simulink model "untitled"  (R2023b)
settings: Solver=FixedStepAuto  StartTime=0.0  StopTime=20  FixedStep=1e-5  MinStep=1e-6  RelTol=1e-3  AbsTol=1e-3
libraries: C_uF_lib x4, nesl_utility x2, SignalEditorBlockLib x1
settings Model: Creator=malli  LastModifiedBy=mavap
settings SolverCC: AutoScaleAbsTol=off  InitialStep=1e-6  MaxConsecutiveMinStep=1000000  AlgebraicLoopSolver=TrustRegion  SolverResetMethod=Robust  EnableFixedStepZeroCrossing=on  MaxZcPerStep=1
settings DataIOCC: MaxDataPoints=1000000  InspectSignalLogs=on
settings DebuggingCC: UnconnectedInputMsg=warning  UnconnectedOutputMsg=warning  UnconnectedLineMsg=warning  SymbolicDimsDataTypeCodeGenerationDiagnostic=none
settings HardwareCC: ProdBitPerLong=64  ProdHWDeviceType=Intel->x86-64 (Linux 64)
settings ModelReferenceCC: EnableRefExpFcnMdlSchedulingChecks=on
settings SFSimCC: CustomCodeUndefinedFunction=UseInterfaceOnly
settings RTWCC: DLArmComputeVersion=19.05
settings SimscapeCC: SimscapeNormalizeSystem=off  SimscapeLogType=all  SimscapeLogSimulationStatistics=on  SimscapeLogToSDI=on  SimscapeLogLimitData=off  SimscapeLogDataHistory=10000000

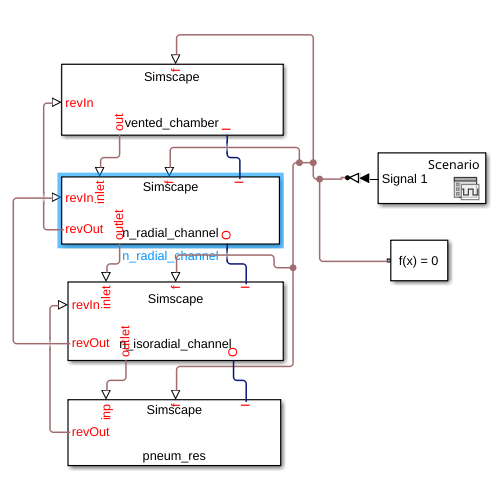
[thumbnail: Simulink's stored preview of the top-level diagram]
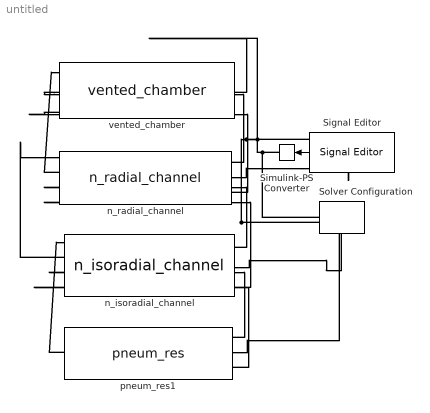
== system untitled ==
  Signal Editor : SignalEditorBlockLib/Signal Editor  FileName=/home/mavap/Documents/MATLAB/C_uF_lumped/Velocity profiles/up10down10.mat  ActiveScenario=Scenario  ActiveSignal=Signal 1  IsBus=off  OutputBusObjectStr=Bus: BusObject  SampleTime=0.00001  ZeroCross=off  OutputAfterFinalValue=Extrapolation  Unit=Hz  PreserveSignalName=on  ApplySigPropsToAllScenarios=on  ApplySigPropsToAllSignals=off
  Simulink-PS Converter : nesl_utility/Simulink-PS Converter  PhysicalDomain=network_engine_domain  SubClassName=ps_input  LeftPortType=input  RightPortType=output  PseudoPeriodic=off  Frequencies=[]  NoiseDistribution=none  NoiseParameters=[]  Unit=Hz  AffineConversion=on  FilteringAndDerivatives=filter  SimscapeFilterOrder=1  InputFilterTimeConstant=0.00001  UdotUserProvided=0
  Solver Configuration : nesl_utility/Solver Configuration  PhysicalDomain=network_engine_domain  SubClassName=solver  LeftPortType=input  RightPortType=generic  Tones=[]  Harmonics=[]  SimulateNoise=off  Profile=off  UseLocalSampling=off  EnableSwitchedLinearOptims=on  FrequencyDomain=off  UseCCode=off  RelTol=0.001  AbsTol=0.001  MinStep=1e-09  ToWorkspace=off  RevertToSquareIcSolve=off  NumHomotopyIterations=100  PhasorMode=off  PhasorModeNumHarmonics=1  ConsistencySolver=NEWTON_XTOL_AFTER_FTOL  IndexReductionMethod=DerivativeReplacement  DoDC=on  ResidualTolerance=1e-09  ConsistencyTolSource=GLOBAL  ConsistencyAbsTol=0.001  ConsistencyRelTol=0.001  ConsistencyTolFactor=0.000001  UseLocalSolver=off  LocalSolverChoice=NE_BACKWARD_EULER_ADVANCER  ResolveIndetEquations=on  FunctionEvalNumThread=1  LocalSolverSampleTime=0.001  DoFixedCost=off  MaxNonlinIter=3  MaxModeIter=2  ComputeImpulses=off  ImpulseIterations=2  LinearAlgebra=auto  LinearAlgebraNumThread=0  EquationFormulation=NE_TIME_EF  DelaysMemoryBudget=1024  AutomaticFiltering=on  FilteringTimeConstant=0.00001  PartitionStorageMethod=AS_NEEDED  PartitionMemoryBudget=1024  PartitionMethod=ROBUST  MultibodyUseLocalSolver=off  MultibodyLocalSolverChoice=ODE1  MultibodyLocalSolverSampleTime=0.001
  n_isoradial_channel : C_uF_lib/n_isoradial_channel  w=2 mm  d=40 um  l=20 mm  r=70 mm  init_fill=0  theta=pi/2  dir=-1  q_specify=off  q_priority=None  q=0 mm^3/s  q_nominal_specify=off  q_nominal_unit=mm^3/s  q_nominal_value=1  q_dot_specify=off  q_dot_priority=None  q_dot=0 mm^3/s^2  q_dot_nominal_specify=off  q_dot_nominal_unit=mm^3/s^2  q_dot_nominal_value=1  f_dot_specify=off  f_dot_priority=None  f_dot=0 Hz/s  f_dot_nominal_specify=off  f_dot_nominal_unit=Hz/s  f_dot_nominal_value=1  p_specify=off  p_priority=None  p=0 Pa  p_nominal_specify=off  p_nominal_unit=Pa  p_nominal_value=1  fill_specify=off  fill_priority=None  fill=0  fill_nominal_specify=off  fill_nominal_unit=1  fill_nominal_value=1  V_liquid_specify=off  V_liquid_priority=None  V_liquid=0 mm^3  V_liquid_nominal_specify=off  V_liquid_nominal_unit=mm^3  V_liquid_nominal_value=1  InO_specify=off  InO_priority=None  InO=0  InO_nominal_specify=off  InO_nominal_unit=1  InO_nominal_value=1  p_IRRF_specify=off  p_IRRF_priority=None  p_IRRF=0 Pa  p_IRRF_nominal_specify=off  p_IRRF_nominal_unit=Pa  p_IRRF_nominal_value=1  p_Euler_specify=off  p_Euler_priority=None  p_Euler=0 Pa  p_Euler_nominal_specify=off  p_Euler_nominal_unit=Pa  p_Euler_nominal_value=1  p_visc_specify=off  p_visc_priority=None  p_visc=0 Pa  p_visc_nominal_specify=off  p_visc_nominal_unit=Pa  p_visc_nominal_value=1  p_cap_specify=off  p_cap_priority=None  p_cap=0 Pa  p_cap_nominal_specify=off  p_cap_nominal_unit=Pa  p_cap_nominal_value=1  wet_specify=off  wet_priority=None  wet=0  wet_nominal_specify=off  wet_nominal_unit=1  wet_nominal_value=1
      settings: InternalSimscapePortConfiguration="{\"Bottom\":[{\"id\":\"O\",\"label\":\"O\",\"type\":\"C_uF.C_uF\"},{\"id\":\"outlet\",\"label\":\"outlet\",\"type\":\"output\"}],\"Left\":[],\"Right\":[{\"id\":\"revIn\",\"label\":\"revIn\",\"type\":\"input\"},{\"id\":\"revOut\",\"label\":\"revOut\",\"type\":\"output\"}],\"Top\":[{\"id\":\"I\",\"label\":\"I\",\"type\":\"C_uF.C_uF\"},{\"id\":\"f\",\"label\":\"f\",\"type\":\"input\"},{\"id\":\"inlet\",\"label\":\"inlet\",\"type\":\"input\"}]}"
  n_radial_channel : C_uF_lib/n_radial_channel  w=2 mm  d=40 um  r_in=20 mm  r_out=70 mm  init_fill=0  theta=pi/2  q_specify=off  q_priority=None  q=0 mm^3/s  q_nominal_specify=off  q_nominal_unit=mm^3/s  q_nominal_value=1  q_dot_specify=off  q_dot_priority=None  q_dot=0 mm^3/s^2  q_dot_nominal_specify=off  q_dot_nominal_unit=mm^3/s^2  q_dot_nominal_value=1  p_specify=off  p_priority=None  p=0 Pa  p_nominal_specify=off  p_nominal_unit=Pa  p_nominal_value=1  fill_specify=off  fill_priority=None  fill=0  fill_nominal_specify=off  fill_nominal_unit=1  fill_nominal_value=1  V_liquid_specify=off  V_liquid_priority=None  V_liquid=0 mm^3  V_liquid_nominal_specify=off  V_liquid_nominal_unit=mm^3  V_liquid_nominal_value=1  InO_specify=off  InO_priority=None  InO=0  InO_nominal_specify=off  InO_nominal_unit=1  InO_nominal_value=1  p_IRRF_specify=off  p_IRRF_priority=None  p_IRRF=0 Pa  p_IRRF_nominal_specify=off  p_IRRF_nominal_unit=Pa  p_IRRF_nominal_value=1  p_cent_specify=off  p_cent_priority=None  p_cent=0 Pa  p_cent_nominal_specify=off  p_cent_nominal_unit=Pa  p_cent_nominal_value=1  p_visc_specify=off  p_visc_priority=None  p_visc=0 Pa  p_visc_nominal_specify=off  p_visc_nominal_unit=Pa  p_visc_nominal_value=1  p_cap_specify=off  p_cap_priority=None  p_cap=0 Pa  p_cap_nominal_specify=off  p_cap_nominal_unit=Pa  p_cap_nominal_value=1  wet_specify=off  wet_priority=None  wet=0  wet_nominal_specify=off  wet_nominal_unit=1  wet_nominal_value=1
      settings: InternalSimscapePortConfiguration="{\"Bottom\":[{\"id\":\"O\",\"label\":\"O\",\"type\":\"C_uF.C_uF\"},{\"id\":\"outlet\",\"label\":\"outlet\",\"type\":\"output\"}],\"Left\":[],\"Right\":[{\"id\":\"revIn\",\"label\":\"revIn\",\"type\":\"input\"},{\"id\":\"revOut\",\"label\":\"revOut\",\"type\":\"output\"}],\"Top\":[{\"id\":\"I\",\"label\":\"I\",\"type\":\"C_uF.C_uF\"},{\"id\":\"f\",\"label\":\"f\",\"type\":\"input\"},{\"id\":\"inlet\",\"label\":\"inlet\",\"type\":\"input\"}]}"
  pneum_res1 : C_uF_lib/pneum_res  G=0  init_fill=0  V_total=300 mm^3  l=10 mm  dist_to_cent=70 mm  p_specify=off  p_priority=None  p=0 Pa  p_nominal_specify=off  p_nominal_unit=Pa  p_nominal_value=1  q_specify=off  q_priority=None  q=0 mm^3/s  q_nominal_specify=off  q_nominal_unit=mm^3/s  q_nominal_value=1  h_liquid_specify=off  h_liquid_priority=None  h_liquid=0 mm  h_liquid_nominal_specify=off  h_liquid_nominal_unit=mm  h_liquid_nominal_value=1  p_cent_specify=off  p_cent_priority=None  p_cent=0 Pa  p_cent_nominal_specify=off  p_cent_nominal_unit=Pa  p_cent_nominal_value=1  f_dot_specify=off  f_dot_priority=None  f_dot=0 Hz/s  f_dot_nominal_specify=off  f_dot_nominal_unit=Hz/s  f_dot_nominal_value=1  p_Euler_specify=off  p_Euler_priority=None  p_Euler=0 Pa  p_Euler_nominal_specify=off  p_Euler_nominal_unit=Pa  p_Euler_nominal_value=1  V_liquid_specify=off  V_liquid_priority=None  V_liquid=0 mm^3  V_liquid_nominal_specify=off  V_liquid_nominal_unit=mm^3  V_liquid_nominal_value=1  fill_specify=off  fill_priority=None  fill=0  fill_nominal_specify=off  fill_nominal_unit=1  fill_nominal_value=1  p_pneum_specify=off  p_pneum_priority=None  p_pneum=0 Pa  p_pneum_nominal_specify=off  p_pneum_nominal_unit=Pa  p_pneum_nominal_value=1
      settings: InternalSimscapePortConfiguration="{\"Bottom\":[],\"Left\":[],\"Right\":[{\"id\":\"revOut\",\"label\":\"revOut\",\"type\":\"output\"}],\"Top\":[{\"id\":\"I\",\"label\":\"I\",\"type\":\"C_uF.C_uF\"},{\"id\":\"f\",\"label\":\"f\",\"type\":\"input\"},{\"id\":\"inp\",\"label\":\"inp\",\"type\":\"input\"}]}"
  vented_chamber : C_uF_lib/vented_chamber  G=0  init_fill=1  V_total=280 mm^3  l=10 mm  dist_to_cent=10 mm  theta=pi / 2  p_specify=off  p_priority=None  p=0 Pa  p_nominal_specify=off  p_nominal_unit=Pa  p_nominal_value=1  q_specify=off  q_priority=None  q=0 mm^3/s  q_nominal_specify=off  q_nominal_unit=mm^3/s  q_nominal_value=1  h_liquid_specify=off  h_liquid_priority=None  h_liquid=0 mm  h_liquid_nominal_specify=off  h_liquid_nominal_unit=mm  h_liquid_nominal_value=1  p_cent_specify=off  p_cent_priority=None  p_cent=0 Pa  p_cent_nominal_specify=off  p_cent_nominal_unit=Pa  p_cent_nominal_value=1  f_dot_specify=off  f_dot_priority=None  f_dot=0 Hz/s  f_dot_nominal_specify=off  f_dot_nominal_unit=Hz/s  f_dot_nominal_value=1  p_Euler_specify=off  p_Euler_priority=None  p_Euler=0 Pa  p_Euler_nominal_specify=off  p_Euler_nominal_unit=Pa  p_Euler_nominal_value=1  V_liquid_specify=off  V_liquid_priority=None  V_liquid=0 mm^3  V_liquid_nominal_specify=off  V_liquid_nominal_unit=mm^3  V_liquid_nominal_value=1  fill_specify=off  fill_priority=None  fill=0  fill_nominal_specify=off  fill_nominal_unit=1  fill_nominal_value=1
      settings: InternalSimscapePortConfiguration="{\"Bottom\":[{\"id\":\"I\",\"label\":\"I\",\"type\":\"C_uF.C_uF\"},{\"id\":\"out\",\"label\":\"out\",\"type\":\"output\"}],\"Left\":[],\"Right\":[{\"id\":\"revIn\",\"label\":\"revIn\",\"type\":\"input\"}],\"Top\":[{\"id\":\"f\",\"label\":\"f\",\"type\":\"input\"}]}"
  wires:
  Signal Editor/1 -> Simulink-PS Converter/1
  connections:
  Simulink-PS Converter/RConn1 -- n_isoradial_channel/LConn2 -- pneum_res1/LConn2 -- n_radial_channel/LConn2 -- vented_chamber/LConn1 -- Solver Configuration/RConn1
  vented_chamber/RConn2 -- n_radial_channel/LConn1
  n_radial_channel/RConn2 -- vented_chamber/RConn1
  vented_chamber/RConn3 -- n_radial_channel/LConn3
  n_isoradial_channel/RConn3 -- pneum_res1/LConn1
  n_radial_channel/RConn3 -- n_isoradial_channel/LConn1
  n_radial_channel/RConn4 -- n_isoradial_channel/LConn3
  n_isoradial_channel/RConn2 -- n_radial_channel/RConn1
  pneum_res1/RConn1 -- n_isoradial_channel/RConn1
  n_isoradial_channel/RConn4 -- pneum_res1/LConn3
